simulink model "FM_System"  (R2024a)
settings: Solver=VariableStepAuto  StartTime=0.0  StopTime=10.0  RelTol=1e-3
undefined symbols (not defined in the file): DiscIntNeverNeededParam
libraries: dspfdesign x1
settings Model: Creator=alice  LastModifiedBy=alice

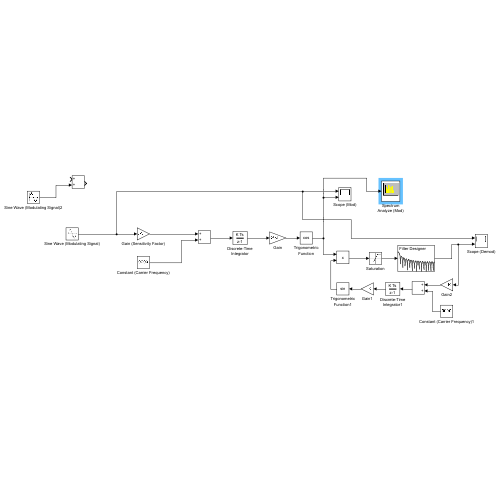
[thumbnail: Simulink's stored preview of the top-level diagram]
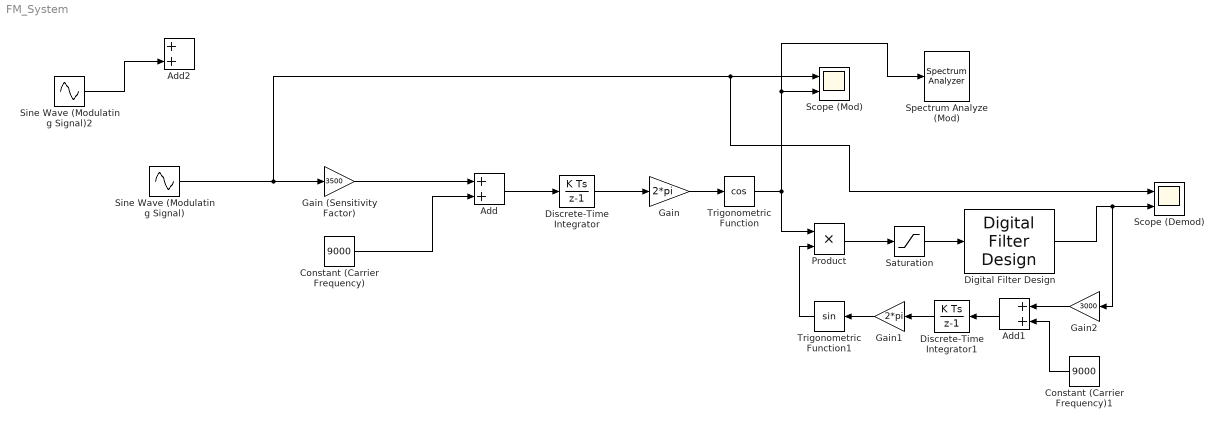
== system FM_System ==
  Add : Sum
  Add1 : Sum
  Add2 : Sum
  Constant (Carrier Frequency) : Constant  Value=9000
  Constant (Carrier Frequency)1 : Constant  Value=9000
  Digital Filter Design : dspfdesign/Digital Filter Design  mwdsp_browser_bugfix_var=off
  Discrete-Time Integrator : DiscreteIntegrator  SampleTime=1e-6  ICPrevOutput=DiscIntNeverNeededParam  ICPrevScaledInput=DiscIntNeverNeededParam
  Discrete-Time Integrator1 : DiscreteIntegrator  SampleTime=1e-6  ICPrevOutput=DiscIntNeverNeededParam  ICPrevScaledInput=DiscIntNeverNeededParam
  Gain : Gain  Gain=2*pi
  Gain (Sensitivity Factor) : Gain  Gain=3500
  Gain1 : Gain  Gain=2*pi
  Gain2 : Gain  Gain=3000
  Product : Product
  Saturation : Saturate
  Scope (Demod) : Scope  NumInputPorts=2
  Scope (Mod) : Scope  NumInputPorts=2
  Sine Wave (Modulating Signal) : Sin  SineType=Sample based  Samples=100  SampleTime=1e-6
  Sine Wave (Modulating Signal)2 : Sin  SineType=Sample based  Amplitude=2  Samples=1000  SampleTime=1e-6
  Spectrum Analyze (Mod) : SpectrumAnalyzer  WindowPosition=[1.000000,49.000000,1280.000000,729.000000,]  ScopeFrameLocation=window  RBW=3  Span=1000000  StartFrequency=-500000  StopFrequency=500000  YLimits=[-254.96952678,54.66463623]  SelectedToolstripTab=spectrumAnalyzerToolstrip.channelMeasurementsTab
  Trigonometric Function : Trigonometry  Operator=cos
  Trigonometric Function1 : Trigonometry
  wires:
  Sine Wave (Modulating Signal)/1 -> Scope (Demod)/1, Scope (Mod)/1, Gain (Sensitivity Factor)/1
  Gain (Sensitivity Factor)/1 -> Add/1
  Constant (Carrier Frequency)/1 -> Add/2
  Add/1 -> Discrete-Time Integrator/1
  Discrete-Time Integrator/1 -> Gain/1
  Gain/1 -> Trigonometric Function/1
  Trigonometric Function/1 -> Spectrum Analyze (Mod)/1, Scope (Mod)/2, Product/1
  Product/1 -> Saturation/1
  Saturation/1 -> Digital Filter Design/1
  Gain1/1 -> Trigonometric Function1/1
  Discrete-Time Integrator1/1 -> Gain1/1
  Add1/1 -> Discrete-Time Integrator1/1
  Gain2/1 -> Add1/1
  Constant (Carrier Frequency)1/1 -> Add1/2
  Digital Filter Design/1 -> Gain2/1, Scope (Demod)/2
  Trigonometric Function1/1 -> Product/2
  Sine Wave (Modulating Signal)2/1 -> Add2/2
